simulink model "PruebaSDRTX"  (R2025b)
settings: Solver=VariableStepAuto  StartTime=0.0  StopTime=inf  RelTol=1e-3
undefined symbols (not defined in the file): img_tx
libraries: commdigbbndpm3 x1, commfilt2 x1, commsdrhw_v2 x1
settings Model: Creator=juand  LastModifiedBy=JuanDiego

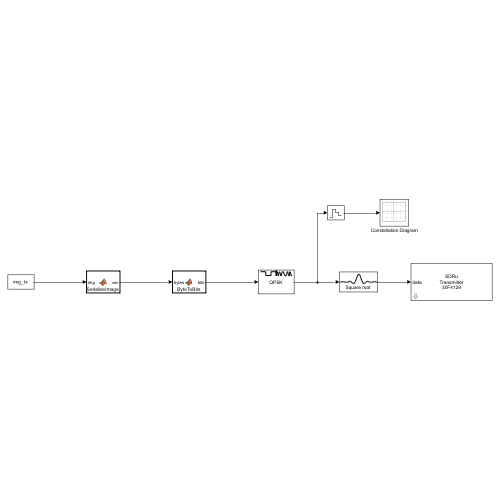
[thumbnail: Simulink's stored preview of the top-level diagram]
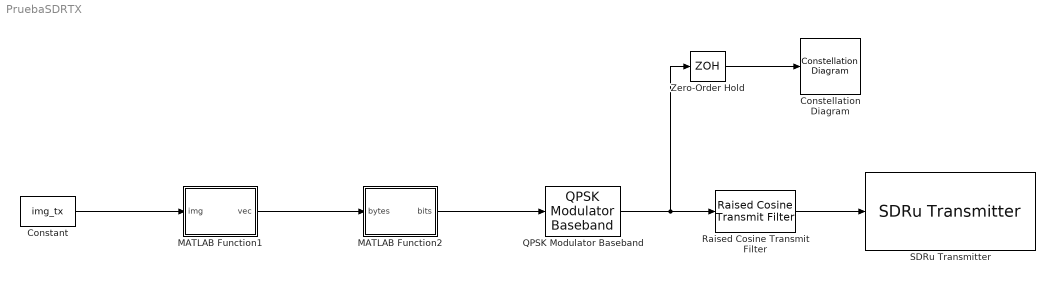
== system PruebaSDRTX ==
  Constant : Constant  Value=img_tx
  Constellation Diagram : ConstellationDiagram  WindowPosition=[1175.000000,267.000000,600.000000,600.000000,]  Visible=on  ScopeFrameLocation=window  SymbolsToDisplaySource=Property  SymbolsToDisplay=5000  ReferenceConstellation=QPSK  ShowReferenceConstellation=off
  MATLAB Function1 : MATLAB Function  TreatAsAtomicUnit=on
  MATLAB Function2 : MATLAB Function  TreatAsAtomicUnit=on
  QPSK Modulator Baseband : commdigbbndpm3/QPSK Modulator Baseband  InType=Bit  Enc=Gray  Ph=pi/4  outDtype=double  outWordLen=16  outUDDataType=sfix(16)  outFracLenMode=Best precision  outFracLen=15  outDataTypeStr=double  outLastDataTypeStr=double
  Raised Cosine Transmit Filter : commfilt2/Raised Cosine Transmit Filter  filtType=Square root  R=0.25  filtSpan=8  N=8  filterGain=1  InputProcessing=Columns as channels (frame based)  RateOptions=Enforce single-rate processing  framing=Mute  checkCoeff=off  variableName=rcTxFilt  checkGain=Normalized  sampMode=Mute  saveAsFlag=0  currentFiltSpan=10  D=(10)/2  launchFVT=on  roundingMode=Floor  overflowMode=off  coeffDataTypeStr=Inherit: Same word length as input  coeffMin=[]  coeffMax=[]  coeffLastDataTypeStr=Inherit: Same word length as input  outputDataTypeStr=Inherit: Same as accumulator  outputMin=[]  outputMax=[]  outputLastDataTypeStr=Inherit: Same as accumulator
  SDRu Transmitter : commsdrhw_v2/SDRu Transmitter  rxtx=tx  initializeIPAddress=0  devMap=0  USRP2_IP=192.168.10.2  USRP_IP_X300=192.168.10.2  USRP_IP_X310=192.168.10.2  USRP_IP_N300=No devices found  USRP_IP_N310=192.168.10.2  USRP_IP_N320=No devices found  USRP_IP_E320=No devices found  USRP_IP_X410=No devices found  USRP_serialNumB200=3136D21  USRP_serialNumB210=30F4129  platform=B210  prevPlatform=B210  lastIPAddressPopup=192.168.10.2  USRP_ID=30F4129  LastIPAddress=192.168.10.2  ChannelMapping=1  centerFrequencySrc=Dialog  centerFrequency=0.9e9  loOffsetSrc=Dialog  loOffset=0  gainSrc=Dialog  gain=50  PPSSource=Internal  clockSource=Internal  EnableGPSLock=off  EnsureSyncGPSTime=off  EnableTimeTrigger=off  triggerTime=5  enableMIMOCableSync=off  EnableRefLock=off  masterClkRateParam=32000000  masterClkRateB200=32e6  masterClkRateB210=32e6  masterClkRateX300=200e6  masterClkRateX310=200e6  masterClkRateN300=125e6  masterClkRateN310=125e6  masterClkRateN320=200e6  masterClkRateE320=30.72e6  masterClkRateX410=250e6  decimInterpSrc=Dialog  lastDecimSource=Dialog  decimInterp=16  USRP2_IP_NUM=[51 48 70 52 49 50 57]  frameLength=362  sampleRate=2000000  TransportDataType=int16  outputDatatype=Same as transport data type  overrunUnderrunPort=off  sampleTime=5.12e-06  dboardInfo=|  HOST_DATA_PORT=30000  HOST_CONTROL_PORT=30001  USRP2_DATA_PORT=32769  USRP2_CONTROL_PORT=32768  bufferMode=Continuous streaming  EnableBurstMode=off  NumFramesInBurst=100
      | dbid: 0
      |           dbName: 'no db found'
      |          freqMin: 0
      |          freqMax: 0
      |          gainMin: 0
      |          gainMax: 0
      |     gainStepSize: 0
  Zero-Order Hold : ZeroOrderHold
  wires:
  Constant/1 -> MATLAB Function1/1(img)
  MATLAB Function1/1(vec) -> MATLAB Function2/1(bytes)
  MATLAB Function2/1(bits) -> QPSK Modulator Baseband/1
  Raised Cosine Transmit Filter/1 -> SDRu Transmitter/1
  QPSK Modulator Baseband/1 -> Zero-Order Hold/1, Raised Cosine Transmit Filter/1
  Zero-Order Hold/1 -> Constellation Diagram/1

== matlab function PruebaSDRTX/MATLAB Function2 ==
  data: bytes input; bits output
function bits = ByteToBits(bytes)

bits_matrix = de2bi(bytes,8,'left-msb');

bits = bits_matrix(:);

end

== matlab function PruebaSDRTX/MATLAB Function1 ==
  data: img input; vec output
function vec = SerializeImage(img)

vec = reshape(img,[],1);

end
